simulink library "INT_AccPed_DrvDemStpLim"  (R2016b)
settings: Solver=VariableStepAuto  StartTime=0.0  StopTime=10.0  RelTol=1e-3
settings Model: Creator=Administrator  LastModifiedBy=Administrator

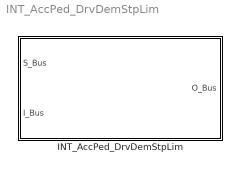
== system INT_AccPed_DrvDemStpLim ==
  INT_AccPed_DrvDemStpLim : Subsystem

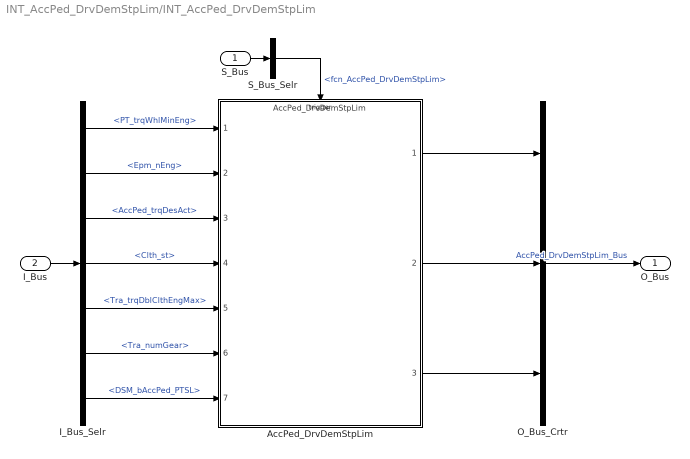
== system INT_AccPed_DrvDemStpLim/INT_AccPed_DrvDemStpLim ==
  S_Bus : Inport
  I_Bus : Inport  Port=2
  AccPed_DrvDemStpLim : ModelReference  ModelNameDialog=AccPed_DrvDemStpLim  SimulationMode=Normal  ModelReferenceVersion=1.7  TriggerPortName=function  TriggerPortTriggerType=function-call  TriggerPortStatesWhenEnabling=held
  I_Bus_Selr : BusSelector  OutputSignals=PT_trqWhlMinEng,Epm_nEng,AccPed_trqDesAct,Clth_st,Tra_trqDblClthEngMax,Tra_numGear,DSM_bAccPed_PTSL
  O_Bus_Crtr : BusCreator  Inputs=3
  S_Bus_Selr : BusSelector  OutputSignals=fcn_AccPed_DrvDemStpLim
  O_Bus : Outport
  wires:
  S_Bus_Selr/1 -> AccPed_DrvDemStpLim/Trigger  "<fcn_AccPed_DrvDemStpLim>"
  S_Bus/1 -> S_Bus_Selr/1
  I_Bus/1 -> I_Bus_Selr/1
  I_Bus_Selr/1 -> AccPed_DrvDemStpLim/1  "<PT_trqWhlMinEng>"
  I_Bus_Selr/2 -> AccPed_DrvDemStpLim/2  "<Epm_nEng>"
  I_Bus_Selr/3 -> AccPed_DrvDemStpLim/3  "<AccPed_trqDesAct>"
  I_Bus_Selr/4 -> AccPed_DrvDemStpLim/4  "<Clth_st>"
  I_Bus_Selr/5 -> AccPed_DrvDemStpLim/5  "<Tra_trqDblClthEngMax>"
  I_Bus_Selr/6 -> AccPed_DrvDemStpLim/6  "<Tra_numGear>"
  I_Bus_Selr/7 -> AccPed_DrvDemStpLim/7  "<DSM_bAccPed_PTSL>"
  O_Bus_Crtr/1 -> O_Bus/1  "AccPed_DrvDemStpLim_Bus"
  AccPed_DrvDemStpLim/1 -> O_Bus_Crtr/1
  AccPed_DrvDemStpLim/2 -> O_Bus_Crtr/2
  AccPed_DrvDemStpLim/3 -> O_Bus_Crtr/3
